simulink model "MPCisnm"  (R2023a)
settings: Solver=ode4  StartTime=0.0  StopTime=tsim  FixedStep=baseRate  RelTol=1e-6  AbsTol=1e-6
values from neighbouring files (symbols this model uses):
  ALGORITHM = 6    [Run_Initializer.m]
  con0 = [n*N, 2*N, N, N, N]    [Run_Initializer.m]
  Gamma1_el = 0.12    [Run_Initializer.m]
  Gamma1_sh = 0.005    [Run_Initializer.m]
  Gamma1_wr = 0.025    [Run_Initializer.m]
  Gamma2_el = 5    [Run_Initializer.m]
  Gamma2_sh = 5    [Run_Initializer.m]
  Gamma2_wr = 5    [Run_Initializer.m]
  Gamma3_el = 10    [Run_Initializer.m]
  Gamma3_sh = 40    [Run_Initializer.m]
  Gamma3_wr = 40    [Run_Initializer.m]
  Gamma4_el = 0.039    [Run_Initializer.m]
  Gamma4_sh = 0.015    [Run_Initializer.m]
  Gamma4_wr = 0.029    [Run_Initializer.m]
  Gamma5_el = 800    [Run_Initializer.m]
  Gamma5_sh = 800    [Run_Initializer.m]
  Gamma5_wr = 800    [Run_Initializer.m]
  Gamma6_el = 0.000001    (= 1e-06)    [Run_Initializer.m]
  Gamma6_sh = 0.005    [Run_Initializer.m]
  Gamma6_wr = 0.02    [Run_Initializer.m]
  init_states_BLACK = [ct;thetat0].'    [Run_Initializer.m]
  init_states_BLUE = [pobj1;0].'    [Run_Initializer.m]
  init_states_RED = xi(1:3).'    [Run_Initializer.m]
  Kd_elarm = 0.8    [Run_Initializer.m]
  Kd_sharm = 1.0    (= 1)    [Run_Initializer.m]
  Kd_wrarm = 0.6    [Run_Initializer.m]
  Kp_elarm = 1.2    [Run_Initializer.m]
  Kp_sharm = 1.5    [Run_Initializer.m]
  Kp_wrarm = 2    [Run_Initializer.m]
  maxiterations = 10    [Run_Initializer.m]
  N = 15    [Run_Initializer.m]    (also in theFastMPCSolver2.m = length(z)/9)
  Phi = 2*H + kappa*P.'*d2*P    [theFastMPCSolver2.m]
  Td = 2    [Run_Initializer.m]
  thetat_dot = 2.5 * d2r    (= 0.0436332312999)    [Run_Initializer.m]
  tol = 0.00015    [Run_Initializer.m]
  Tz_lim_elarm = .1    (= 0.1)    [Run_Initializer.m]
  Tz_lim_sharm = .1    (= 0.1)    [Run_Initializer.m]
  Tz_lim_wrarm = .1    (= 0.1)    [Run_Initializer.m]
  vobj1 = [0.00;0.00]    [Run_Initializer.m]
  vtar = [-0.005;0.005]    [Run_Initializer.m]
undefined symbols (not defined in the file or in its folder): a1, a2, a3, Ad, b0, b1, b2, b3, baseRate, cdockdeltax, cdockoa, Cmat, DiscIntNeverNeededParam, drop_states_ARM, drop_states_BLACK, drop_states_BLUE, drop_states_RED, ecoa, F_Black_X_nominal, F_Black_Y_nominal, F_Blue_X_nominal, F_Blue_Y_nominal, F_red_X_nominal, F_red_Y_nominal, F_thrusters_BLACK, F_thrusters_BLUE, F_thrusters_RED, Fmat, gamma, H, IBLACK, IBLUE, IDIST, IEE, IPROX, IRED, Kd_tb, Kd_tblue, Kd_tr, Kd_xb, Kd_xblue, Kd_xr, Kd_yb, Kd_yblue, Kd_yr, KOZ_actual, Kp_tb, Kp_tblue, Kp_tr, Kp_xb, Kp_xblue, Kp_xr, Kp_yb, Kp_yblue, Kp_yr, mBLACK, mBLUE, mDIST, mEE, mPROX ... (+31)
libraries: nvidiaSharedBlocks x8, simulink x8, dspsigops x6, dspstat3 x5, MainLibrary x4
(part 9 of 10)

== matlab function MPCisnm/Simulate Plant Dynamics/RED and ARM Dynamics/RED + ARM/RED + ARM Dynamics/Coriolis Function1 ==
  data: a1 parameter; a2 parameter; a3 parameter; b0 parameter; b1 parameter; b2 parameter; mPROX parameter; mDIST parameter; mEE parameter; Phi parameter; CoriolisS output; x input
function CoriolisS = CoriolisFunc3LINK(a1,a2,a3,b0,b1,b2,mPROX,mDIST,mEE,Phi,x)
%CORIOLISFUNC3LINK
%    CORIOLISS = CORIOLISFUNC3LINK(A1,A2,A3,B0,B1,B2,mPROX,mDIST,mEE,PHI,Q0,Q1,Q2,Q3,Q0_DOT,Q1_DOT,Q2_DOT,Q3_DOT)

%    This function was generated by the Symbolic Math Toolbox version 8.0.
%    05-Nov-2017 11:48:44

q0 = x(3);
q1 = x(4);
q2 = x(5);
q3 = x(6);

q0_dot = x(9);
q1_dot = x(10);
q2_dot = x(11);
q3_dot = x(12);

t2 = a1+b1;
t3 = a1.*mPROX;
t4 = mDIST.*t2;
t5 = mEE.*t2;
t6 = t3+t4+t5;
t7 = a2.*mDIST;
t8 = a2+b2;
t9 = mEE.*t8;
t10 = t7+t9;
t11 = pi.*(1.0./2.0);
t12 = q0_dot.*t6;
t13 = q1_dot.*t6;
t14 = q0+q1+t11;
t15 = cos(t14);
t16 = t12+t13;
t17 = q0_dot.*t10;
t18 = q1_dot.*t10;
t19 = q2_dot.*t10;
t20 = q0+q1+q2+t11;
t21 = cos(t20);
t22 = t17+t18+t19;
t23 = a3.*mEE.*q0_dot;
t24 = a3.*mEE.*q1_dot;
t25 = a3.*mEE.*q2_dot;
t26 = a3.*mEE.*q3_dot;
t27 = q0+q1+q2+q3+t11;
t28 = cos(t27);
t29 = t23+t24+t25+t26;
t30 = b0.*mPROX;
t31 = b0.*mDIST;
t32 = b0.*mEE;
t33 = t30+t31+t32;
t34 = (pi/2-Phi)+q0;
t35 = sin(t14);
t36 = sin(t20);
t37 = sin(t27);
t38 = q0_dot+q1_dot+q2_dot+q3_dot;
t39 = q0+q1+q2+q3;
t40 = a1.*b0.*mPROX.*q1_dot;
t41 = a1.*b0.*mDIST.*q1_dot;
t42 = a1.*b0.*mEE.*q1_dot;
t43 = b0.*b1.*mDIST.*q1_dot;
t44 = b0.*b1.*mEE.*q1_dot;
t45 = (pi/2-Phi)-q1;
t46 = cos(t45);
t47 = a2.*b0.*mDIST.*q1_dot;
t48 = a2.*b0.*mDIST.*q2_dot;
t49 = a2.*b0.*mEE.*q1_dot;
t50 = a2.*b0.*mEE.*q2_dot;
t51 = b0.*b2.*mEE.*q1_dot;
t52 = b0.*b2.*mEE.*q2_dot;
t53 = -(pi/2-Phi)+q1+q2;
t54 = cos(t53);
t55 = a3.*b0.*mEE.*q1_dot;
t56 = a3.*b0.*mEE.*q2_dot;
t57 = a3.*b0.*mEE.*q3_dot;
t58 = -(pi/2-Phi)+q1+q2+q3;
t59 = cos(t58);
t60 = a2.*b1.*mDIST.*q2_dot;
t61 = a1.*b2.*mEE.*q2_dot;
t62 = a2.*b1.*mEE.*q2_dot;
t63 = b1.*b2.*mEE.*q2_dot;
t64 = a1.*a2.*mDIST.*q2_dot;
t65 = a1.*a2.*mEE.*q2_dot;
t66 = sin(q2);
t67 = t60+t61+t62+t63+t64+t65;
t68 = a3.*b2.*mEE.*q3_dot;
t69 = a2.*a3.*mEE.*q3_dot;
t70 = sin(q3);
t71 = t68+t69;
t72 = a3.*b1.*mEE.*q2_dot;
t73 = a3.*b1.*mEE.*q3_dot;
t74 = a1.*a3.*mEE.*q2_dot;
t75 = a1.*a3.*mEE.*q3_dot;
t76 = q2+q3;
t77 = sin(t76);
t78 = t72+t73+t74+t75;
t79 = a2.*b0.*mDIST.*q0_dot;
t80 = a2.*b0.*mEE.*q0_dot;
t81 = b0.*b2.*mEE.*q0_dot;
t82 = t47+t48+t49+t50+t51+t52+t79+t80+t81;
t83 = a3.*b0.*mEE.*q0_dot;
t84 = t55+t56+t57+t83;
t85 = a1.*b0.*mPROX.*q0_dot;
t86 = a1.*b0.*mDIST.*q0_dot;
t87 = a1.*b0.*mEE.*q0_dot;
t88 = b0.*b1.*mDIST.*q0_dot;
t89 = b0.*b1.*mEE.*q0_dot;
t90 = a2.*b1.*mDIST.*q0_dot;
t91 = a1.*b2.*mEE.*q0_dot;
t92 = a2.*b1.*mDIST.*q1_dot;
t93 = a2.*b1.*mEE.*q0_dot;
t94 = a1.*b2.*mEE.*q1_dot;
t95 = a2.*b1.*mEE.*q1_dot;
t96 = b1.*b2.*mEE.*q0_dot;
t97 = b1.*b2.*mEE.*q1_dot;
t98 = a1.*a2.*mDIST.*q0_dot;
t99 = a1.*a2.*mDIST.*q1_dot;
t100 = a1.*a2.*mEE.*q0_dot;
t101 = a1.*a2.*mEE.*q1_dot;
t102 = t60+t61+t62+t63+t64+t65+t90+t91+t92+t93+t94+t95+t96+t97+t98+t99+t100+t101;
t103 = a3.*b1.*mEE.*q0_dot;
t104 = a3.*b1.*mEE.*q1_dot;
t105 = a1.*a3.*mEE.*q0_dot;
t106 = a1.*a3.*mEE.*q1_dot;
t107 = t72+t73+t74+t75+t103+t104+t105+t106;
t108 = t79+t80+t81;
t109 = t54.*t108;
t110 = t59.*t83;
t111 = t90+t91+t92+t93+t94+t95+t96+t97+t98+t99+t100+t101;
t112 = t66.*t111;
t113 = t103+t104+t105+t106;
t114 = t77.*t113;
t115 = a2.*q0_dot;
t116 = a2.*q1_dot;
t117 = a2.*q2_dot;
t118 = b2.*q0_dot;
t119 = b2.*q1_dot;
t120 = b2.*q2_dot;
t121 = t115+t116+t117+t118+t119+t120;
t122 = a3.*mEE.*t70.*t121;
t123 = a1.*q0_dot;
t124 = a1.*q1_dot;
t125 = b1.*q0_dot;
t126 = b1.*q1_dot;
t127 = t123+t124+t125+t126;
t128 = a3.*mEE.*t77.*t127;
CoriolisS = reshape([0.0,0.0,0.0,0.0,0.0,0.0,0.0,0.0,0.0,0.0,0.0,0.0,-t15.*t16-t21.*t22-t28.*t29-q0_dot.*t33.*cos(t34),-t16.*t35-t22.*t36-t29.*t37-q0_dot.*t33.*sin(t34),-t66.*t67-t70.*t71-t77.*t78-t46.*(t40+t41+t42+t43+t44)-t59.*(t55+t56+t57)-t54.*(t47+t48+t49+t50+t51+t52),t109+t110-t66.*t67-t70.*t71-t77.*t78+t46.*(t85+t86+t87+t88+t89),t109+t110+t112+t114-t70.*t71,t110+t122+t128,-t15.*t16-t21.*t22-t28.*t29,-t16.*t35-t22.*t36-t29.*t37,-t66.*t67-t54.*t82-t70.*t71-t59.*t84-t77.*t78-t46.*(t40+t41+t42+t43+t44+t85+t86+t87+t88+t89),-t66.*t67-t70.*t71-t77.*t78,t112+t114-t70.*t71,t122+t128,-t21.*t22-t28.*t29,-t22.*t36-t29.*t37,-t54.*t82-t70.*t71-t59.*t84-t66.*t102-t77.*t107,-t70.*t71-t66.*t102-t77.*t107,-a3.*mEE.*q3_dot.*t8.*t70,a3.*mEE.*t8.*t70.*(q0_dot+q1_dot+q2_dot),a3.*mEE.*t38.*sin(t39),-a3.*mEE.*t38.*cos(t39),-a3.*b0.*mEE.*t38.*t59-a3.*mEE.*t8.*t38.*t70-a3.*mEE.*t2.*t38.*t77,-a3.*mEE.*t8.*t38.*t70-a3.*mEE.*t2.*t38.*t77,-a3.*mEE.*t8.*t38.*t70,0.0],[6,6]);
end

== matlab function MPCisnm/Triggered Subsystem/MATLAB Function ==
  data: xi input; CONTROL output; x0 input; rhold input; ct input; pobj1 input; vtar input; vobj1 input; thetat0 input; thetat_dot input; x0 output; rhold output; CPUTIME output; pdockr parameter; rdock parameter; Ad parameter; con0 parameter; Cmat parameter; Umat parameter; Fmat parameter; H parameter; gamma parameter; tol parameter; Td parameter; N parameter; thetah parameter; KOZ_actual parameter; Sj parameter; rcone parameter; ALGORITHM parameter; umax parameter; taumax parameter; n parameter; pdockoa parameter; ecoa parameter; cdockoa parameter; maxiterations parameter; cdockdeltax parameter
function [CONTROL, x0, rhold, CPUTIME] = MPC(xi,x0, rhold, ct, pobj1, vtar, vobj1, thetat0, thetat_dot, pdockr, rdock, Ad, con0, Cmat, Umat, Fmat, H, gamma, tol, Td, N, thetah, KOZ_actual, Sj, rcone, ALGORITHM, umax, taumax, n, pdockoa, ecoa, cdockoa, maxiterations, cdockdeltax)
    % COPY-PASTED FROM LOOP IN MAIN
    d2r = pi/180;
    
    N = 15;
    maxiterations = 10;
    
    % The moving target and obstacle positions for the current sampling instant, k
    [pobj1hz, ptar] = theMovingObstacleHorizonParameters(Td,N,ct,pobj1,vtar,vobj1);
    
    % The rotating target parameters for the current sampling instant, k
    [thetat,m1,m2,nc1,nc2,pdock,xt,cdock] = theRotatingTargetHorizonParameters(Td,N,ptar,vtar,pdockr,rhold,rdock,cdockoa,pdockoa,ecoa,thetat_dot,thetah,thetat0,cdockdeltax);
       
    % Reshape the xt variable for use in theObjectiveFunction, ignore the
    % current state and reform into [03 xt(2) 03 xt(2) 03 ... 03 xt(N+1)]
    xt9 = zeros(9,N);
    xt9(4:9,:) = xt(:,2:N+1);
    xt9 = reshape(xt9, [9*N,1]);
    
    % The reference trajectory of the chaser over the horizon of instant k
    pxref = theReferenceTrajectory(x0,N); % 2xN

    % The points ro on the KOZ boundaries of the obstacles over the horizon
    ro_1 = theObstacleLinearizer(pxref,pobj1hz(:,2:N+1),KOZ_actual);
    ro_t = theObstacleLinearizer(pxref,ptar(:,2:N+1),rhold);
    
    % Reshape pdock for use in the linearized matrix constraints
    pdock9 = zeros(9,N);
    pdock9(4:5,:) = pdock(:,2:N+1);
    pdock9 = reshape(pdock9, [9*N,1]);

    % Make the ro_X and robj9 vectors for obstacle constraints
    ro_1_9 = zeros(9,N);
    ro_1_9(4:5,:) = ro_1;
    ro_1_9 = reshape(ro_1_9,9*N,1);

    ro_t_9 = zeros(9,N);
    ro_t_9(4:5,:) = ro_t;
    ro_t_9 = reshape(ro_t_9,9*N,1);

    robj1_9 = zeros(9,N);
    robj1_9(4:5,:) = pobj1hz(:,2:N+1);
    robj1_9 = reshape(robj1_9,9*N,1);

    rtar_9 = zeros(9,N);
    rtar_9(4:5,:) = ptar(:,2:N+1);
    rtar_9 = reshape(rtar_9,9*N,1);

    % Make the matrix for obstacle constraints
    S1 = Sj;
    St = [1/(rhold*rhold), 0; 0, 1/(rhold*rhold)];

    E1 = (ro_1 - pobj1hz(:,2:N+1)).' * S1;
    Et = (ro_t - ptar(:,2:N+1)).' * St;

    D1 = zeros(N,(9*N));
    Dt = zeros(N,(9*N));
    for row = 1:N
        D1(row,4+(row-1)*9:5+(row-1)*9) = E1(row,:);
        Dt(row,4+(row-1)*9:5+(row-1)*9) = Et(row,:);
    end  
    
    % Define the b vector for Cx = b dynamics constraint
    bvec = zeros(6*N,1);
    bvec(1:6) = Ad*xi;
    
    % Define arrays for the hyperplane normal arrays to be used for the entry cone constraints
    nc1m = zeros(N,9*N);
    nc2m = zeros(N,9*N);
        
    % Determine if the entry cone constraints should be on
    if ((xi(1:2) - cdock(1:2,1)).' * (xi(1:2) - cdock(1:2,1)) < rcone*rcone) % if chaser is within rcone range
        
        temp1 = -nc1(2,:) * x0(4:5) + nc1(2,:) * pdock9(4:5);
        temp2 = nc2(2,:) * x0(4:5) - nc2(2,:) * pdock9(4:5);
        
              
        if temp1 <= 0 && temp2 <= 0 % only turn ec constraints on if it won't cause infeasibilities at the next step
            
        
            withEntryCone = 1; % turn on
            con = [n*N, 2*N, N, N, N, N, N];

            % Create Nx2N matrix of the entry cone normal to each hyperplane
            % Should be in the form
            % ncm = [ 0_1x3 n1_1x2 0_1x4 0_1x3  0_1x2 0_1x4  ... 0_1x3 0_1x2 0_1x4
            %         0_1x3  0_1x2 0_1x4 0_1x3 n2_1x2 0_1x4  ... 0_1x3 0_1x2 0_1x4
            %                           ...
            %         0_1x3  0_1x2 0_1x4 0_1x3  0_1x2 0_1x4  ... 0_1x3 nN+1_1x2 0_1x4
            for i=1:N
                nc1m(i,4+(i-1)*9:5+(i-1)*9) = nc1(i+1,:);
                nc2m(i,4+(i-1)*9:5+(i-1)*9) = nc2(i+1,:);
            end
        else
            
            withEntryCone = 0; % turn off
            con = con0;

            % FOR PLOTTING PURPOSES
            m1 = NaN;
            m2 = NaN;
        end
                
    else
        withEntryCone = 0; % turn off
        con = con0;
        
        % FOR PLOTTING PURPOSES
        m1 = NaN;
        m2 = NaN;
    end
    

    
%     if ALGORITHM == 5     
        % Constraint Matrix
        % if ~withEntryCone
        %     Wmat = [-2*D1;-2*Dt];
        % else
        %     Wmat = [-2*D1;-2*Dt;-nc1m;nc2m];
        % end
%     % THIS NEEDS TO BE CLEANED UP
%     elseif ALGORITHM == 6 || ALGORITHM == 7
        if withEntryCone
            Wmat = zeros(10*N,9*N);
            hvec = zeros(10*N,1);
        else
            Wmat = zeros(8*N,9*N);
            hvec = zeros(8*N,1);
        end

        for index = 0:N-1
            blockc = 9*index;
            if withEntryCone
                blockr = 10*index;
                Wmat(9+blockr,:) = -nc1m(index+1,:);
                Wmat(10+blockr,:) = nc2m(index+1,:);
            else
                blockr = 8*index;
            end
            Wmat(1+blockr:3+blockr,1+blockc:3+blockc) = eye(3);
            Wmat(4+blockr:6+blockr,1+blockc:3+blockc) = -eye(3);
            Wmat(7+blockr,:) = -2*D1(index+1,:);
            Wmat(8+blockr,:) = -2*Dt(index+1,:);
        end

        f_D1 = -ones(N,1) - D1*(ro_1_9 + robj1_9);
        f_Dt = -ones(N,1) - Dt*(ro_t_9 + rtar_9);   
        f_ec1 = zeros(N,1);
        f_ec2 = zeros(N,1);
        if withEntryCone % if entry cone constraints turned on
            f_ec1 = -nc1m * pdock9;
            f_ec2 = nc2m * pdock9;
        end

        for index = 0:N-1
            if withEntryCone % if entry cone constraints turned on
                blockr = 10*index;
                hvec(9+blockr) = f_ec1(index+1);
                hvec(10+blockr) = f_ec2(index+1);
            else
                blockr = 8*index;
            end

            hvec(1+blockr:3+blockr) = [umax;umax;taumax];
            hvec(4+blockr:6+blockr) = [umax;umax;taumax];
            hvec(7+blockr) = f_D1(index+1);
            hvec(8+blockr) = f_Dt(index+1);
        end
% 
%     end
    
    % Constraint upper and lower limits
%     if ALGORITHM == 5
        % [cl,cu,bineqvec] = theConstraintLimits4(Umat,Fmat,Wmat,con0,con,...
        %     D1,Dt,ro_1_9,ro_t_9,robj1_9,rtar_9,nc1m,...
        %     nc2m,pdock9);
%     end
    
    

%     
%     % Ensure a feasible start
%     if ALGORITHM == 6 || ALGORITHM == 7
%         if any((hvec - Wmat*x0) <= 0)
%             disp('Started with infeasible solution (outside).');
%             infeas0 = find((hvec - Wmat*x0) <= 0);
%             disp(infeas0)
% 
%             % Find a new feasible z-val for the violated constraint(s)
%             for ind = infeas0.'
%                 if size(con) == size(con0) % no ec constraints yet
%                     ind_startrange = 7 + 8*idivide(ind,int16(8+1));
%                     ind_endrange = ind_startrange + 1;
%                 else
%                     ind_startrange = 7 + 10*idivide(ind,int16(10+1));
%                     ind_endrange = ind_startrange + 3;
%                 end
% %                 disp(ind_startrange)
% %                 disp(ind_endrange)
%                     
%                 z_infeas_ind = find(Wmat(ind,:)); % optimization variable(s) to vary
%     %             disp('z(infeas)=')
%     %             disp(z_infeas_ind)
% 
%                 newind = z_infeas_ind - 9;
%                 
%                 search_range = 1;
%                 search_stepnum = 1001;
%                 
%                 while (1)
%                     if newind < 0
%                         disp("Sampling...")
% 
%                         % make a grid of search points
%                         try_x = linspace(x0(z_infeas_ind(1))-search_range,x0(z_infeas_ind(1))+search_range,search_stepnum);
%                         try_y = linspace(x0(z_infeas_ind(2))-search_range,x0(z_infeas_ind(2))+search_range,search_stepnum);
%                         [xx,yy] = meshgrid(try_x,try_y);
% 
%                         % calcuate the constraint at each grid point
% %                         temp = zeros(search_stepnum,search_stepnum);
%                         temp2 = zeros(search_stepnum*search_stepnum,3);
%                         for i1=1:search_stepnum
%                             for i2 = 1:search_stepnum
%                                 temp = hvec(ind_startrange:ind_endrange) - Wmat(ind_startrange:ind_endrange,z_infeas_ind)*[xx(i1,i2);yy(i1,i2)];
% 
%                                 % take note of grid points that satisfy the constraint
%                                 if ~any(temp <= 0)
%                                     temp2((i1-1)*search_stepnum+i2,1) = min(temp);
%                                     temp2((i1-1)*search_stepnum+i2,2) = i1;
%                                     temp2((i1-1)*search_stepnum+i2,3) = i2;
%                                 end
%                             end
%                         end
% 
%                         % get rid of data that does not satisfy the constraints
%                         temp2( ~any(temp2,2), : ) = [];  %rows
%                         
%                         if isempty(temp2)
%                             search_range = 3;
%                             search_stepnum = search_stepnum * 2;
%                             continue
%                         end
% 
%                         % choose one of the grid points that satisfy the constraint
%                         % currently finds the first minimum value... could be further improved
%                         ind_of_min = find(temp2(:,1) == min(temp2(:,1)));
%                         ind_chosen = ind_of_min(1);
% 
%                         % update the x0 with the new grid point
%                         [i1i2_chosen] = temp2(ind_chosen,[2,3]);
%                         i1_chosen = i1i2_chosen(1);
%                         i2_chosen = i1i2_chosen(2);
%                         x0(z_infeas_ind) = [xx(i1_chosen,i2_chosen);yy(i1_chosen,i2_chosen)];                     
%                         
%                     else
%                         x0(z_infeas_ind) = x0(newind); % re-tracing previous sol'n
%                     end
% 
%                     if (hvec(ind)- Wmat(ind,:)*x0) <= 0
%                         if newind < 0
%                             disp("Solution not in sample range.")
%                         else
%                             newind = newind - 9;
%                         end
%                     else
%                         disp("Resolved.")
%                         break
%                         
%                     end
%                 end
%             end
%         end
%        
%     end
%     
%     
%     
%     % Setup Options
%     if ALGORITHM == 5
        % options = optimoptions('quadprog','Algorithm','active-set','MaxIterations',10);
%     elseif ALGORITHM == 6 || ALGORITHM == 7
        nu = zeros(6*N,1);
%     end
%     
%     % Solve!
%     if ALGORITHM == 5
        % tic
        % [x,fval] = quadprog(H,-H.'*xt9,Wmat,bineqvec,Cmat,bvec,cl,cu,x0,options);
        % CPUTIME = toc;
%     elseif ALGORITHM == 6
%         disp('----------------------------------------------')
%         disp(string(count))
%         
        tic
        [x,nu] = theFastMPCSolver2(x0,nu,xt9,H,Cmat,bvec,Wmat,hvec,1e-9,0.01,0.95,maxiterations);
        CPUTIME = toc;
%     elseif ALGORITHM == 7
%         disp('----------------------------------------------')
%         disp(string(count))
%         tic
%         [x,nu] = theFastMPCSolver3(x0,nu,xt9,H,Cmat,bvec,Wmat,hvec,1e-9,0.01,0.95,maxiterations);
%         solCPUtime = toc;
%     end
   

    % Save data
%     sol(end+1:end+9) = x(1:9);
%     soliter(1:n,count) = xi;
%     soliter(n+1:n+9*N,count) = x;
%     solpobj(count,1) = pobj1hz(1,1); 
%     solpobj(count,2) = pobj1hz(2,1);
%     solpobj(count,3) = pobj2hz(1,1);
%     solpobj(count,4) = pobj2hz(2,1);
%     solptar(count,1) = ptar(1,1);
%     solptar(count,2) = ptar(2,1);
%     solm1(count,1) = m1(1);
%     solm2(count,1) = m2(1);
%     solthetat(count,1) = thetat(1);
%     solpdock(count,1:2) = pdock(:,1);
%     if ALGORITHM == 0
%         solJ(end+1) = theObjectiveFunction0(x,N,xt,P,Q,R);
%     elseif ALGORITHM > 0
%         solJ(end+1) = theObjectiveFunction123(x,xt9,H);
%     end
%     count = count + 1;

    CONTROL = x(1:3);
    
    % Determine if the chaser is docked using the 'current' positions of
    % the chaser and docking condition; done using only position
    if (xi(1:2) - cdock(1:2,1)).' * (xi(1:2) - cdock(1:2,1)) < tol
        isdocked = 1;
    end
    
    % Update rhold if:
    %  - the position of the chaser matches the holding position, within tolerance
    %  - the attitude of the chaser matches the docking condition, within tolerance
    %  - the holding radius is larger than its minimum allowable size, rdock
    if abs((xi(1:2) - xt(1:2,1)).' * (xi(1:2) - xt(1:2,1))) < 0.5 % if position error is below tolerance
        if abs(xi(3) - cdock(3,1)) < 10*d2r % if attitude error is below tolerance
            if rhold > rdock
                rhold = rhold * gamma; % decrease the holding radius
                if rhold < rdock
                    rhold = rdock; % set to the minimum holding radius, rdock
                end
            end
        end
    end
    
    % Set the next guess as the solution from the previous iteration
    xi = x(4:9); % the next 'current' state of the chaser spacecraft
    % x0 = [x(10:end);0;0;0;Ad*x0(4+9*(N-2):9+9*(N-2)) + Bd*x0(1+9*(N-1):3+9*(N-1))];
    x0 = [x(10:end);0;0;0;x(4+9*(N-1):9+9*(N-1))];
        
    % Set the next 'current' target and obstacle positions
%     ct = ptar(:,2);
%     pobj1 = pobj1hz(:,2); 
%     pobj2 = pobj2hz(:,2);
        
    % Set the new target theta value for the next iteration
%     thetat0 = thetat(2);
    
end

== matlab function MPCisnm/Simulate Plant Dynamics/RED and ARM Dynamics/RED + ARM/RED + ARM Dynamics/Inertia Function 1 ==
  data: mRED parameter; IRED parameter; Phi parameter; b0 parameter; a1 parameter; b1 parameter; a2 parameter; b2 parameter; a3 parameter; b3 parameter; mPROX parameter; mDIST parameter; mEE parameter; IPROX parameter; IDIST parameter; InertiaS output; x input; IEE parameter
function InertiaS = InertiaFunc3LINK(mRED, IRED, Phi, b0, a1, b1, a2, b2, a3, b3, mPROX, mDIST, mEE, IPROX, IDIST, x, IEE)

    q0 = x(3);
    q1 = x(4);
    q2 = x(5);
    q3 = x(6);
    
    t2 = a1+b1;
    t3 = a1.*mPROX;
    t4 = mDIST.*t2;
    t5 = mEE.*t2;
    t6 = q0+q1;
    t7 = cos(t6);
    t8 = t3+t4+t5;
    t9 = a2.*mDIST;
    t10 = a2+b2;
    t11 = mEE.*t10;
    t12 = q0+q1+q2;
    t13 = cos(t12);
    t14 = t9+t11;
    t15 = q0+q1+q2+q3;
    t16 = cos(t15);
    t17 = mRED+mPROX+mDIST+mEE;
    t18 = b0.*mPROX;
    t19 = b0.*mDIST;
    t20 = b0.*mEE;
    t21 = t18+t19+t20;
    t22 = (pi/2-Phi)+q0;
    t23 = sin(t6);
    t24 = sin(t12);
    t25 = sin(t15);
    t26 = a2.*mEE;
    t27 = b2.*mEE;
    t28 = t9+t26+t27;
    t29 = sin(t22);
    t86 = t7.*t8;
    t87 = t13.*t14;
    t88 = a3.*mEE.*t16;
    t30 = -t86-t87-t88-t21.*t29;
    t31 = cos(t22);
    t32 = t21.*t31;
    t89 = t8.*t23;
    t90 = t14.*t24;
    t91 = a3.*mEE.*t25;
    t33 = t32-t89-t90-t91;
    t34 = a1.^2;
    t35 = a2.^2;
    t36 = b0.^2;
    t37 = b1.^2;
    t38 = a1.*a2.*mDIST.*2.0;
    t39 = a1.*a2.*mEE.*2.0;
    t40 = a2.*b1.*mDIST.*2.0;
    t41 = a1.*b2.*mEE.*2.0;
    t42 = a2.*b1.*mEE.*2.0;
    t43 = b1.*b2.*mEE.*2.0;
    t44 = t38+t39+t40+t41+t42+t43;
    t45 = cos(q2);
    t46 = t44.*t45;
    t47 = a2.*a3.*mEE.*2.0;
    t48 = a3.*b2.*mEE.*2.0;
    t49 = t47+t48;
    t50 = cos(q3);
    t51 = t49.*t50;
    t52 = a1.*a3.*mEE.*2.0;
    t53 = a3.*b1.*mEE.*2.0;
    t54 = t52+t53;
    t55 = q2+q3;
    t56 = cos(t55);
    t57 = t54.*t56;
    t58 = (pi/2-Phi)-q1;
    t59 = sin(t58);
    t60 = -(pi/2-Phi)+q1+q2;
    t61 = sin(t60);
    t62 = -(pi/2-Phi)+q1+q2+q3;
    t63 = sin(t62);
    t64 = mPROX.*t34;
    t65 = mDIST.*t34;
    t66 = mEE.*t34;
    t67 = mDIST.*t35;
    t68 = mEE.*t35;
    t69 = a3.^2;
    t70 = mEE.*t69;
    t71 = mDIST.*t37;
    t72 = mEE.*t37;
    t73 = b2.^2;
    t74 = mEE.*t73;
    t75 = a1.*b1.*mDIST.*2.0;
    t76 = a1.*b1.*mEE.*2.0;
    t77 = a2.*b2.*mEE.*2.0;
    t78 = a2.*b0.*mDIST;
    t79 = a2.*b0.*mEE;
    t80 = b0.*b2.*mEE;
    t81 = t78+t79+t80;
    t82 = a1.*a3.*mEE;
    t83 = a3.*b1.*mEE;
    t84 = t82+t83;
    t85 = t56.*t84;
    t92 = a1.*b0.*mPROX;
    t93 = a1.*b0.*mDIST;
    t94 = a1.*b0.*mEE;
    t95 = b0.*b1.*mDIST;
    t96 = b0.*b1.*mEE;
    t97 = t92+t93+t94+t95+t96;
    t98 = t59.*t97;
    t112 = t61.*t81;
    t113 = a3.*b0.*mEE.*t63;
    t99 = IPROX+IDIST+IEE+t46+t51+t57+t64+t65+t66+t67+t68+t70+t71+t72+t74+t75+t76+t77+t98-t112-t113;
    t100 = a1.*a2.*mDIST;
    t101 = a1.*a2.*mEE;
    t102 = a2.*b1.*mDIST;
    t103 = a1.*b2.*mEE;
    t104 = a2.*b1.*mEE;
    t105 = b1.*b2.*mEE;
    t106 = t100+t101+t102+t103+t104+t105;
    t107 = t45.*t106;
    t108 = a2.*a3.*mEE;
    t109 = a3.*b2.*mEE;
    t110 = t108+t109;
    t111 = t50.*t110;
    t114 = IDIST+IEE+t51+t67+t68+t70+t74+t77+t85+t107;
    t115 = IEE+t70+t85+t111;
    t116 = IEE+t70+t111;
    InertiaS = reshape([t17,0.0,t30,-t86-t87-t88,-t88-t13.*t28,-t88,0.0,t17,t33,-t89-t90-t91,-t91-t24.*t28,-t91,t30,t33,IRED+IPROX+IDIST+IEE+t46+t51+t57+t64+t65+t66+t67+t68+t70+t71+t72+t74+t75+t76+t77+t59.*(a1.*b0.*mPROX.*2.0+a1.*b0.*mDIST.*2.0+a1.*b0.*mEE.*2.0+b0.*b1.*mDIST.*2.0+b0.*b1.*mEE.*2.0)+mPROX.*t36+mDIST.*t36+mEE.*t36-t61.*(a2.*b0.*mDIST.*2.0+a2.*b0.*mEE.*2.0+b0.*b2.*mEE.*2.0)-a3.*b0.*mEE.*t63.*2.0,t99,IDIST+IEE+t51+t67+t68+t70+t74+t77+t85+t107-t112-t113,IEE+t70+t85+t111-t113,-t7.*t8-t13.*t14-a3.*mEE.*t16,-t8.*t23-t14.*t24-a3.*mEE.*t25,t99,IPROX+IDIST+IEE+t46+t51+t57+t64+t65+t66+t67+t68+t70+t71+t72+t74+t75+t76+t77,t114,t115,-t13.*t28-a3.*mEE.*t16,-t24.*t28-a3.*mEE.*t25,IDIST+IEE+t51+t67+t68+t70+t74+t77+t85+t107-t61.*t81-a3.*b0.*mEE.*t63,t114,IDIST+IEE+t51+t67+t68+t70+t74+t77,t116,-a3.*mEE.*t16,-a3.*mEE.*t25,IEE+t70+t85+t111-a3.*b0.*mEE.*t63,t115,t116,IEE+t70],[6,6]);
end

== matlab function MPCisnm/Phase #3: Experiment/Change RED Behavior/Sub-Phase #1/Hough Control/MATLAB Function2 ==
  data: Oy output; z input; Ox output
function [Oy, Ox]   = C3( z )
%C3 gives the rotation matrix about the z-axis for an angle 'z'
%   z - the angle about the z-axis which you rotate
%   A - the rotation matrix

Ox = [cos(z) sin(z); -sin(z) cos(z)]*[1;0];
Oy = [cos(z) sin(z); -sin(z) cos(z)]*[0;1];
end

== matlab function MPCisnm/Simulate Plant Dynamics/BLACK Dynamics/BLACK Dynamics Model/MATLAB Function ==
  data: control_inputs input; x_ddot output; mBLACK parameter; IBLACK parameter
function x_ddot = BLACK_dynamics(control_inputs, mBLACK, IBLACK)

%#codegen
% Fully define the size of x_ddot() for code generation:
x_ddot     = zeros(3,1);

% Extract the control inputs from the control_input vector:
Fx        = control_inputs(1);              % [N]
Fy        = control_inputs(2);              % [N]
Tz        = control_inputs(3);              % [N.m]

% Calculate the state acceleration vector:
x_ddot(1) = Fx/mBLACK;                      % [m/s^2]
x_ddot(2) = Fy/mBLACK;                      % [m/s^2]
x_ddot(3) = Tz/IBLACK;                      % [rad/s^2]

end

== matlab function MPCisnm/Simulate Plant Dynamics/BLUE Dynamics/BLUE  Dynamics Model/MATLAB Function ==
  data: control_inputs input; x_ddot output; mBLUE parameter; IBLUE parameter
function x_ddot = BLUE_dynamics(control_inputs, mBLUE, IBLUE)%#codegen
% Fully define the size of x_ddot() for code generation:
x_ddot     = zeros(3,1);

% Extract the control inputs from the control_input vector:
Fx        = control_inputs(1);              % [N]
Fy        = control_inputs(2);              % [N]
Tz        = control_inputs(3);              % [N.m]

% Calculate the state acceleration vector:
x_ddot(1) = Fx/mBLUE;                      % [m/s^2]
x_ddot(2) = Fy/mBLUE;                      % [m/s^2]
x_ddot(3) = Tz/IBLUE;                      % [rad/s^2]

end

== matlab function MPCisnm/Simulate Plant Dynamics/BLUE Dynamics/Sample and Hold Data to Match PhaseSpace (BLUE)/MATLAB Function ==
  data: TIME input; y output; SERVER input
function y = fcn(TIME, SERVER)

if mod(TIME,SERVER) == 0
    y = 1;
else
    y = 0;
end

== matlab function MPCisnm/Simulate Plant Dynamics/RED and ARM Dynamics/RED Only/RED Dynamics/RED Dynamics Model/MATLAB Function ==
  data: control_inputs input; x_ddot output; mRED parameter; IRED parameter
    function x_ddot = RED_dynamics(control_inputs, mRED, IRED)
    
        %#codegen
        % Fully define the size of x_ddot() for code generation:
        x_ddot     = zeros(3,1);
        
        % Extract the servicer model parameters from the model_param vector defined
        % in initialize.m:
        
        % Extract the control inputs from the control_input vector:
        Fx        = control_inputs(1);              % [N]
        Fy        = control_inputs(2);              % [N]
        Tz        = control_inputs(3);              % [N.m]
        
        % Calculate the state acceleration vector:
        x_ddot(1) = Fx/mRED;                      % [m/s^2]
        x_ddot(2) = Fy/mRED;                      % [m/s^2]
        x_ddot(3) = Tz/IRED;                      % [rad/s^2]
    
    end

== matlab function MPCisnm/Simulate Plant Dynamics/BLACK Dynamics/Sample and Hold Data to Match PhaseSpace (BLACK)/MATLAB Function ==
  data: TIME input; y output; SERVER input
function y = fcn(TIME, SERVER)

if mod(TIME,SERVER) == 0
    y = 1;
else
    y = 0;
end

== matlab function MPCisnm/Simulate Plant Dynamics/RED and ARM Dynamics/RED Only/RED Dynamics/Sample and Hold Data to Match PhaseSpace (RED)/MATLAB Function ==
  data: TIME input; y output; SERVER input
function y = fcn(TIME, SERVER)

if mod(TIME,SERVER) == 0
    y = 1;
else
    y = 0;
end

== matlab function MPCisnm/Thruster Control Code/Change BLACK Behavior/Calculate Thruster ON//OFF/MATLAB Function ==
  data: H output; thruster_dist2CG_BLACK parameter; F_thrusters_BLACK parameter
function H = MakeH(thruster_dist2CG_BLACK,F_thrusters_BLACK)

Vec1 = [ -1
         -1
          0 
          0
          1
          1
          0
          0 ];
      
Vec2 = [  0
          0
          1
          1
          0
          0
         -1
         -1 ];
     
Vec3 = thruster_dist2CG_BLACK./1000;

Mat1 = [Vec1, Vec2, Vec3]';

Mat2 = diag((F_thrusters_BLACK./2));

H    = Mat1*Mat2;

end

== matlab function MPCisnm/Thruster Control Code/Change BLACK Behavior/Calculate Thruster ON//OFF/MATLAB Function1 ==
  data: H output; thruster_dist2CG_BLACK parameter; F_thrusters_BLACK parameter
function H = MakeH(thruster_dist2CG_BLACK,F_thrusters_BLACK)

Vec1 = [ -1
         -1
          0 
          0
          1
          1
          0
          0 ];
      
Vec2 = [  0
          0
          1
          1
          0
          0
         -1
         -1 ];
     
Vec3 = thruster_dist2CG_BLACK./1000;

Mat1 = [Vec1, Vec2, Vec3]';

Mat2 = diag((F_thrusters_BLACK));

H    = Mat1*Mat2;

end

== matlab function MPCisnm/Thruster Control Code/Change BLACK Behavior/Calculate Thruster ON//OFF/MATLAB Function2 ==
  data: ThrustPer_Final output; ThrustPer input
function ThrustPer_Final  = ThrusterSat(ThrustPer)

ValveTime       = 0.007;
TControl        = 0.1;
ThrustPer_Final = zeros(8,1);

if max(ThrustPer) > 1
    ThrustPer_Sat = ThrustPer/max(ThrustPer);
else
    ThrustPer_Sat = ThrustPer;
end

for i = 1:8
    if ThrustPer_Sat(i) > ValveTime/TControl 
        ThrustPer_Final(i) = ThrustPer_Sat(i);
    else
        ThrustPer_Final(i) = 0;
    end
end
   

end

== matlab function MPCisnm/Thruster Control Code/Change BLACK Behavior/Calculate Thruster ON//OFF/Rotate Forces to Inertial/Create Rotation Matrix ==
  data: Rz input; C_Ib output
function C_Ib = RotateFrame(Rz)

C_bI = [  cos(Rz) sin(Rz)
         -sin(Rz) cos(Rz) ];

C_Ib = inv(C_bI);

end

== matlab function MPCisnm/Thruster Control Code/Change BLACK Behavior/Rotate Forces to Body/Create Rotation Matrix ==
  data: Rz input; C_bI output
function C_bI = RotateFrame(Rz)

C_bI = [  cos(Rz) sin(Rz)
         -sin(Rz) cos(Rz) ];

end

== matlab function MPCisnm/Thruster Control Code/Change BLUE Behavior/Calculate Thruster ON//OFF/MATLAB Function ==
  data: H output; thruster_dist2CG_BLUE parameter; F_thrusters_BLUE parameter
function H = MakeH(thruster_dist2CG_BLUE,F_thrusters_BLUE)

Vec1 = [ -1
         -1
          0 
          0
          1
          1
          0
          0 ];
      
Vec2 = [  0
          0
          1
          1
          0
          0
         -1
         -1 ];
     
Vec3 = thruster_dist2CG_BLUE./1000;

Mat1 = [Vec1, Vec2, Vec3]';

Mat2 = diag((F_thrusters_BLUE./2));

H    = Mat1*Mat2;

end

== matlab function MPCisnm/Thruster Control Code/Change BLUE Behavior/Calculate Thruster ON//OFF/MATLAB Function1 ==
  data: H output; thruster_dist2CG_BLUE parameter; F_thrusters_BLUE parameter
function H = MakeH(thruster_dist2CG_BLUE,F_thrusters_BLUE)

Vec1 = [ -1
         -1
          0 
          0
          1
          1
          0
          0 ];
      
Vec2 = [  0
          0
          1
          1
          0
          0
         -1
         -1 ];
     
Vec3 = thruster_dist2CG_BLUE./1000;

Mat1 = [Vec1, Vec2, Vec3]';

Mat2 = diag((F_thrusters_BLUE./2));

H    = Mat1*Mat2;

end

== matlab function MPCisnm/Thruster Control Code/Change BLUE Behavior/Calculate Thruster ON//OFF/MATLAB Function2 ==
  data: ThrustPer_Final output; ThrustPer input
function ThrustPer_Final  = ThrusterSat(ThrustPer)

ValveTime       = 0.007;
TControl        = 0.1;
ThrustPer_Final = zeros(8,1);

if max(ThrustPer) > 1
    ThrustPer_Sat = ThrustPer/max(ThrustPer);
else
    ThrustPer_Sat = ThrustPer;
end

for i = 1:8
    if ThrustPer_Sat(i) > ValveTime/TControl 
        ThrustPer_Final(i) = ThrustPer_Sat(i);
    else
        ThrustPer_Final(i) = 0;
    end
end
   

end

== matlab function MPCisnm/Thruster Control Code/Change BLUE Behavior/Calculate Thruster ON//OFF/Rotate Forces to Inertial/Create Rotation Matrix ==
  data: Rz input; C_Ib output
function C_Ib = RotateFrame(Rz)

C_bI = [  cos(Rz) sin(Rz)
         -sin(Rz) cos(Rz) ];

C_Ib = inv(C_bI);

end

== matlab function MPCisnm/Thruster Control Code/Change BLUE Behavior/Rotate Forces to Body/Create Rotation Matrix ==
  data: Rz input; C_bI output
function C_bI = RotateFrame(Rz)

C_bI = [  cos(Rz) sin(Rz)
         -sin(Rz) cos(Rz) ];

end

== matlab function MPCisnm/Phase #2: Initial Position/Change BLACK Behavior/Hough Control/MATLAB Function2 ==
  data: Oy output; z input; Ox output
function [Oy, Ox]   = C3( z )
%C3 gives the rotation matrix about the z-axis for an angle 'z'
%   z - the angle about the z-axis which you rotate
%   A - the rotation matrix

Ox = [cos(z) sin(z); -sin(z) cos(z)]*[1;0];
Oy = [cos(z) sin(z); -sin(z) cos(z)]*[0;1];
end

== matlab function MPCisnm/Phase #2: Initial Position/Change BLACK Behavior/Hough Control/MATLAB Function3 ==
  data: z input; Ox output
function Ox    = C3( z )
%C3 gives the rotation matrix about the z-axis for an angle 'z'
%   z - the angle about the z-axis which you rotate
%   A - the rotation matrix

Ox = [cos(z) sin(z); -sin(z) cos(z)]*[1;0];
end

== matlab function MPCisnm/Phase #2: Initial Position/Change BLACK Behavior/Hough Control/MATLAB Function4 ==
  data: Oy input; e_out output; e_in input
function e_out = fcn(Oy, e_in)

a = sign(Oy'*e_in);
e_out = -a*norm(e_in);

== matlab function MPCisnm/Phase #2: Initial Position/Change BLUE Behavior/Hough Control/MATLAB Function2 ==
  data: Oy output; z input; Ox output
function [Oy, Ox]   = C3( z )
%C3 gives the rotation matrix about the z-axis for an angle 'z'
%   z - the angle about the z-axis which you rotate
%   A - the rotation matrix

Ox = [cos(z) sin(z); -sin(z) cos(z)]*[1;0];
Oy = [cos(z) sin(z); -sin(z) cos(z)]*[0;1];
end

== matlab function MPCisnm/Thruster Control Code/Change RED Behavior/Rotate Forces to Body/Create Rotation Matrix ==
  data: Rz input; C_bI output
function C_bI = RotateFrame(Rz)

C_bI = [  cos(Rz) sin(Rz)
         -sin(Rz) cos(Rz) ];

end

== matlab function MPCisnm/Phase #2: Initial Position/Change BLUE Behavior/Hough Control/MATLAB Function3 ==
  data: z input; Ox output
function Ox    = C3( z )
%C3 gives the rotation matrix about the z-axis for an angle 'z'
%   z - the angle about the z-axis which you rotate
%   A - the rotation matrix

Ox = [cos(z) sin(z); -sin(z) cos(z)]*[1;0];
end

== matlab function MPCisnm/Phase #2: Initial Position/Change BLUE Behavior/Hough Control/MATLAB Function4 ==
  data: Oy input; e_out output; e_in input
function e_out = fcn(Oy, e_in)

a = sign(Oy'*e_in);
e_out = -a*norm(e_in);

== matlab function MPCisnm/Phase #2: Initial Position/Change RED Behavior/Hough Control/MATLAB Function2 ==
  data: Oy output; z input; Ox output
function [Oy, Ox]   = C3( z )
%C3 gives the rotation matrix about the z-axis for an angle 'z'
%   z - the angle about the z-axis which you rotate
%   A - the rotation matrix

Ox = [cos(z) sin(z); -sin(z) cos(z)]*[1;0];
Oy = [cos(z) sin(z); -sin(z) cos(z)]*[0;1];
end

== matlab function MPCisnm/Phase #2: Initial Position/Change RED Behavior/Hough Control/MATLAB Function3 ==
  data: z input; Ox output
function Ox    = C3( z )
%C3 gives the rotation matrix about the z-axis for an angle 'z'
%   z - the angle about the z-axis which you rotate
%   A - the rotation matrix

Ox = [cos(z) sin(z); -sin(z) cos(z)]*[1;0];
end

== matlab function MPCisnm/Phase #2: Initial Position/Change RED Behavior/Hough Control/MATLAB Function4 ==
  data: Oy input; e_out output; e_in input
function e_out = fcn(Oy, e_in)

a = sign(Oy'*e_in);
e_out = -a*norm(e_in);

== matlab function MPCisnm/Phase #3: Experiment/Change BLACK Behavior/Sub-Phase #4/BLACK_RzD/Wrap1/MATLAB Function ==
  data: u input; wrappedAngle output
function wrappedAngle = wrapAngle(u)

wrappedAngle = atan2(sin(u),cos(u));

end

== matlab function MPCisnm/Phase #3: Experiment/Change BLACK Behavior/Sub-Phase #4/Hough Control/MATLAB Function2 ==
  data: Oy output; z input; Ox output
function [Oy, Ox]   = C3( z )
%C3 gives the rotation matrix about the z-axis for an angle 'z'
%   z - the angle about the z-axis which you rotate
%   A - the rotation matrix

Ox = [cos(z) sin(z); -sin(z) cos(z)]*[1;0];
Oy = [cos(z) sin(z); -sin(z) cos(z)]*[0;1];
end

== matlab function MPCisnm/Phase #3: Experiment/Change BLACK Behavior/Sub-Phase #4/Hough Control/MATLAB Function3 ==
  data: z input; Ox output
function Ox    = C3( z )
%C3 gives the rotation matrix about the z-axis for an angle 'z'
%   z - the angle about the z-axis which you rotate
%   A - the rotation matrix

Ox = [cos(z) sin(z); -sin(z) cos(z)]*[1;0];
end

== matlab function MPCisnm/Phase #3: Experiment/Change BLACK Behavior/Sub-Phase #4/Hough Control/MATLAB Function4 ==
  data: Oy input; e_out output; e_in input
function e_out = fcn(Oy, e_in)

a = sign(Oy'*e_in);
e_out = -a*norm(e_in);

== matlab function MPCisnm/Phase #3: Experiment/Change BLACK Behavior/Sub-Phase #2 /Hough Control/MATLAB Function2 ==
  data: Oy output; z input; Ox output
function [Oy, Ox]   = C3( z )
%C3 gives the rotation matrix about the z-axis for an angle 'z'
%   z - the angle about the z-axis which you rotate
%   A - the rotation matrix

Ox = [cos(z) sin(z); -sin(z) cos(z)]*[1;0];
Oy = [cos(z) sin(z); -sin(z) cos(z)]*[0;1];
end

== matlab function MPCisnm/Phase #3: Experiment/Change BLACK Behavior/Sub-Phase #1/Hough Control/MATLAB Function2 ==
  data: Oy output; z input; Ox output
function [Oy, Ox]   = C3( z )
%C3 gives the rotation matrix about the z-axis for an angle 'z'
%   z - the angle about the z-axis which you rotate
%   A - the rotation matrix

Ox = [cos(z) sin(z); -sin(z) cos(z)]*[1;0];
Oy = [cos(z) sin(z); -sin(z) cos(z)]*[0;1];
end

== matlab function MPCisnm/Phase #3: Experiment/Change BLACK Behavior/Sub-Phase #1/Hough Control/MATLAB Function3 ==
  data: z input; Ox output
function Ox    = C3( z )
%C3 gives the rotation matrix about the z-axis for an angle 'z'
%   z - the angle about the z-axis which you rotate
%   A - the rotation matrix

Ox = [cos(z) sin(z); -sin(z) cos(z)]*[1;0];
end

== matlab function MPCisnm/Phase #3: Experiment/Change BLUE Behavior/Sub-Phase #1/Hough Control/MATLAB Function2 ==
  data: Oy output; z input; Ox output
function [Oy, Ox]   = C3( z )
%C3 gives the rotation matrix about the z-axis for an angle 'z'
%   z - the angle about the z-axis which you rotate
%   A - the rotation matrix

Ox = [cos(z) sin(z); -sin(z) cos(z)]*[1;0];
Oy = [cos(z) sin(z); -sin(z) cos(z)]*[0;1];
end

== matlab function MPCisnm/Phase #3: Experiment/Change BLUE Behavior/Sub-Phase #1/Hough Control/MATLAB Function3 ==
  data: z input; Ox output
function Ox    = C3( z )
%C3 gives the rotation matrix about the z-axis for an angle 'z'
%   z - the angle about the z-axis which you rotate
%   A - the rotation matrix

Ox = [cos(z) sin(z); -sin(z) cos(z)]*[1;0];
end

== matlab function MPCisnm/Phase #3: Experiment/Change BLUE Behavior/Sub-Phase #1/Hough Control/MATLAB Function4 ==
  data: Oy input; e_out output; e_in input
function e_out = fcn(Oy, e_in)

a = sign(Oy'*e_in);
e_out = -a*norm(e_in);

== matlab function MPCisnm/Phase #3: Experiment/Change BLUE Behavior/Sub-Phase #4/Hough Control/MATLAB Function4 ==
  data: Oy input; e_out output; e_in input
function e_out = fcn(Oy, e_in)

a = sign(Oy'*e_in);
e_out = -a*norm(e_in);

== matlab function MPCisnm/Phase #3: Experiment/Change RED Behavior/Sub-Phase #1/Hough Control/MATLAB Function3 ==
  data: z input; Ox output
function Ox    = C3( z )
%C3 gives the rotation matrix about the z-axis for an angle 'z'
%   z - the angle about the z-axis which you rotate
%   A - the rotation matrix

Ox = [cos(z) sin(z); -sin(z) cos(z)]*[1;0];
end

== matlab function MPCisnm/Phase #3: Experiment/Change RED Behavior/Sub-Phase #4/Subsystem/MATLAB Function1 ==
  data: theta_ps input; theta_cont output; theta_psm1 input; revcounter input; revcounter output
function [theta_cont,revcounter]  = fcn(theta_ps,theta_psm1,revcounter)
    
    % Compare the new Rz value to the one previous... has it wrapped?
    if abs(theta_ps-theta_psm1) > 300*pi/180
        % Yes, it has wrapped
            if theta_ps > theta_psm1
                revcounter = revcounter - 1;
            else
                revcounter = revcounter + 1;
            end
    end
    
    theta_cont = theta_ps + revcounter*2*pi;
    
end

== matlab function MPCisnm/Phase #3: Experiment/Change RED Behavior/Sub-Phase #1/Hough Control/MATLAB Function4 ==
  data: Oy input; e_out output; e_in input
function e_out = fcn(Oy, e_in)

a = sign(Oy'*e_in);
e_out = -a*norm(e_in);

== matlab function MPCisnm/Phase #3: Experiment/Change BLUE Behavior/Sub-Phase #2 /Hough Control/MATLAB Function4 ==
  data: Oy input; e_out output; e_in input
function e_out = fcn(Oy, e_in)

a = sign(Oy'*e_in);
e_out = -a*norm(e_in);

== matlab function MPCisnm/Phase #3: Experiment/Change RED Behavior/Sub-Phase #4/Subsystem/MATLAB Function3 ==
  data: theta_ps input; theta_cont output; theta_psm1 input; revcounter input; revcounter output
function [theta_cont,revcounter]  = fcn(theta_ps,theta_psm1,revcounter)
    
    % Compare the new Rz value to the one previous... has it wrapped?
    if abs(theta_ps-theta_psm1) > 300*pi/180
        % Yes, it has wrapped
            if theta_ps > theta_psm1
                revcounter = revcounter - 1;
            else
                revcounter = revcounter + 1;
            end
    end
    
    theta_cont = theta_ps + revcounter*2*pi;
    
end

== matlab function MPCisnm/Phase #3: Experiment/Change BLACK Behavior/Sub-Phase #2 /Hough Control/MATLAB Function3 ==
  data: z input; Ox output
function Ox    = C3( z )
%C3 gives the rotation matrix about the z-axis for an angle 'z'
%   z - the angle about the z-axis which you rotate
%   A - the rotation matrix

Ox = [cos(z) sin(z); -sin(z) cos(z)]*[1;0];
end

== matlab function MPCisnm/Phase #3: Experiment/Change BLACK Behavior/Sub-Phase #2 /Hough Control/MATLAB Function4 ==
  data: Oy input; e_out output; e_in input
function e_out = fcn(Oy, e_in)

a = sign(Oy'*e_in);
e_out = -a*norm(e_in);

== matlab function MPCisnm/Thruster Control Code/Change RED Behavior/Calculate Thruster ON//OFF/MATLAB Function ==
  data: H output; thruster_dist2CG_RED parameter; F_thrusters_RED parameter; theta_1 input; theta_2 input; theta_3 input; mRED parameter; mPROX parameter; mDIST parameter; mEE parameter; Phi parameter; b0 parameter; a1 parameter; b1 parameter; a2 parameter; b2 parameter; a3 parameter; b3 parameter
function H   = MakeHWithArm(thruster_dist2CG_RED,F_thrusters_RED, theta_1, theta_2, theta_3, mRED, mPROX, mDIST, mEE, Phi, b0, a1, b1, a2, b2, a3, b3)
    
    link1_com_x = b0*cos(Phi) + a1*cos(pi/2 + theta_1);
    link1_com_y = b0*sin(Phi) + a1*sin(pi/2 + theta_1);
    
    link2_com_x = link1_com_x + b1*cos(pi/2 + theta_1) + a2*cos(pi/2 + theta_1 + theta_2);
    link2_com_y = link1_com_y + b1*sin(pi/2 + theta_1) + a2*sin(pi/2 + theta_1 + theta_2);
    
    link3_com_x = link2_com_x + b2*cos(pi/2 + theta_1 + theta_2) + a3*cos(pi/2 + theta_1 + theta_2 + theta_3);
    link3_com_y = link2_com_y + b2*sin(pi/2 + theta_1 + theta_2) + a3*sin(pi/2 + theta_1 + theta_2 + theta_3);
    
    delta_com_due_to_arm_x = (mPROX*link1_com_x + mDIST*link2_com_x + mEE*link3_com_x)/(mRED + mPROX + mDIST + mEE)*1000; % [mm]
    delta_com_due_to_arm_y = (mPROX*link1_com_y + mDIST*link2_com_y + mEE*link3_com_y)/(mRED + mPROX + mDIST + mEE)*1000; % [mm]
    
    adjusted_thruster_dist2CG_RED = [thruster_dist2CG_RED(1)-delta_com_due_to_arm_y;
                                     thruster_dist2CG_RED(2)-delta_com_due_to_arm_y;
                                     thruster_dist2CG_RED(3)-delta_com_due_to_arm_x;
                                     thruster_dist2CG_RED(4)-delta_com_due_to_arm_x;
                                     thruster_dist2CG_RED(5)+delta_com_due_to_arm_y;
                                     thruster_dist2CG_RED(6)+delta_com_due_to_arm_y;
                                     thruster_dist2CG_RED(7)+delta_com_due_to_arm_x;
                                     thruster_dist2CG_RED(8)+delta_com_due_to_arm_x];
                                     
    
    
    Vec1 = [ -1
             -1
              0 
              0
              1
              1
              0
              0 ];
          
    Vec2 = [  0
              0
              1
              1
              0
              0
             -1
             -1 ];
         
    Vec3 = adjusted_thruster_dist2CG_RED./1000;
    
    Mat1 = [Vec1, Vec2, Vec3]';
    
    Mat2 = diag((F_thrusters_RED./2));
    
    H    = Mat1*Mat2;

end

== matlab function MPCisnm/Thruster Control Code/Change RED Behavior/Calculate Thruster ON//OFF/MATLAB Function1 ==
  data: H output; thruster_dist2CG_RED parameter; F_thrusters_RED parameter
function H = MakeH(thruster_dist2CG_RED,F_thrusters_RED)

Vec1 = [ -1
         -1
          0 
          0
          1
          1
          0
          0 ];
      
Vec2 = [  0
          0
          1
          1
          0
          0
         -1
         -1 ];
     
Vec3 = thruster_dist2CG_RED./1000;

Mat1 = [Vec1, Vec2, Vec3]';

Mat2 = diag((F_thrusters_RED));

H    = Mat1*Mat2;

end

== matlab function MPCisnm/Thruster Control Code/Change RED Behavior/Calculate Thruster ON//OFF/MATLAB Function2 ==
  data: ThrustPer_Final output; ThrustPer input
function ThrustPer_Final  = ThrusterSat(ThrustPer)

ValveTime       = 0.007;
TControl        = 0.1;
ThrustPer_Final = zeros(8,1);

if max(ThrustPer) > 1
    ThrustPer_Sat = ThrustPer/max(ThrustPer);
else
    ThrustPer_Sat = ThrustPer;
end

for i = 1:8
    if ThrustPer_Sat(i) > ValveTime/TControl 
        ThrustPer_Final(i) = ThrustPer_Sat(i);
    else
        ThrustPer_Final(i) = 0;
    end
end
   

end

== matlab function MPCisnm/Thruster Control Code/Change RED Behavior/Calculate Thruster ON//OFF/Rotate Forces to Inertial/Create Rotation Matrix ==
  data: Rz input; C_Ib output
function C_Ib = RotateFrame(Rz)

C_bI = [  cos(Rz) sin(Rz)
         -sin(Rz) cos(Rz) ];

C_Ib = inv(C_bI);

end

== matlab function MPCisnm/Simulate Plant Dynamics/RED and ARM Dynamics/RED + ARM/RED + ARM Dynamics/Dynamics Model ==
  data: xdot output; x input; InertiaS input; CoriolisS input; u input; Gamma1_sh parameter; Gamma2_sh parameter; Gamma3_sh parameter; Gamma5_sh parameter; Gamma4_sh parameter; Gamma6_sh parameter; Gamma1_el parameter; Gamma2_el parameter; Gamma3_el parameter; Gamma5_el parameter; Gamma4_el parameter; Gamma6_el parameter; Gamma1_wr parameter; Gamma2_wr parameter; Gamma3_wr parameter; Gamma5_wr parameter; Gamma4_wr parameter; Gamma6_wr parameter
function xdot  = DynamicsModel(x, InertiaS, CoriolisS, u,...
    Gamma1_sh, Gamma2_sh, Gamma3_sh, Gamma5_sh, Gamma4_sh, Gamma6_sh,...
    Gamma1_el, Gamma2_el, Gamma3_el, Gamma5_el, Gamma4_el, Gamma6_el,...
    Gamma1_wr, Gamma2_wr, Gamma3_wr, Gamma5_wr, Gamma4_wr, Gamma6_wr)


    fqdot1 = Gamma1_sh*(tanh(Gamma2_sh*x(10)) - tanh(Gamma3_sh*x(10))) + Gamma4_sh*tanh(Gamma5_sh*x(10)) + Gamma6_sh*x(10);

    fqdot2 = Gamma1_el*(tanh(Gamma2_el*x(11)) - tanh(Gamma3_el*x(11))) + Gamma4_el*tanh(Gamma5_el*x(11)) + Gamma6_el*x(11);

    fqdot3 = Gamma1_wr*(tanh(Gamma2_wr*x(12)) - tanh(Gamma3_wr*x(12))) + Gamma4_wr*tanh(Gamma5_wr*x(12)) + Gamma6_wr*x(12);
    
    q_ddot = pinv(InertiaS)*(u - CoriolisS*x(7:12) - [0;0;0;fqdot1;fqdot2;fqdot3]);
    
    xdot   = [ x(7:12)
               q_ddot   ];
           
end

== matlab function MPCisnm/Phase #3: Experiment/Change RED Behavior/Sub-Phase #4/Subsystem/MATLAB Function ==
  data: x input; x output
function x = fcn(x)
    if x > pi
        x  = x - 2*pi;
    elseif x <= -pi
        x = x + 2*pi;
    end
